simulink model "oscilador"  (R2021b)
settings: Solver=VariableStepAuto  StartTime=0.0  StopTime=25.0  RelTol=1e-3
undefined symbols (not defined in the file or in its folder): x10, x20
libraries: simulink x1
settings Model: Creator=Aluno  LastModifiedBy=Aluno

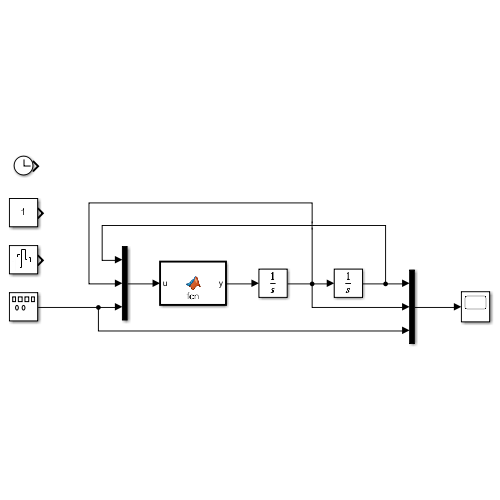
[thumbnail: Simulink's stored preview of the top-level diagram]
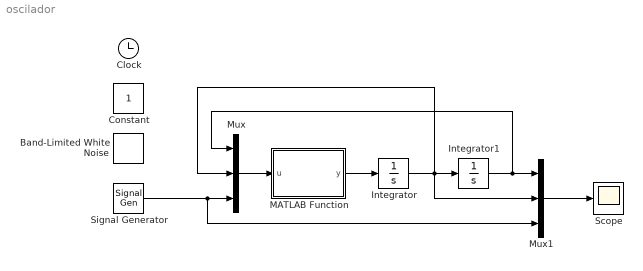
== system oscilador ==
  Band-Limited White Noise : simulink/Sources/Band-Limited White Noise  Cov=[0.1]  Ts=0.1  seed=[23341]
  Clock : Clock
  Constant : Constant
  Integrator : Integrator  InitialCondition=x20
  Integrator1 : Integrator  InitialCondition=x10
  MATLAB Function : MATLAB Function  TreatAsAtomicUnit=on
  Mux : Mux  Inputs=3
  Mux1 : Mux  Inputs=3
  Scope : Scope
  Signal Generator : SignalGenerator  Units=rad/sec
  wires:
  Integrator/1 -> Mux1/2, Mux/2, Integrator1/1
  Integrator1/1 -> Mux/1, Mux1/1
  Mux1/1 -> Scope/1
  Signal Generator/1 -> Mux1/3, Mux/3
  Mux/1 -> MATLAB Function/1(u)
  MATLAB Function/1(y) -> Integrator/1

== matlab function oscilador/MATLAB Function ==
  data: u input; y output
function y = fcn(u)

k = 1;

y = -u(1) + k*u(2) - k*u(1)^2*u(2) + u(3);
